simulink model "distance_tracking"  (R2018b)
settings: Solver=ode8  StartTime=0.0  StopTime=20  FixedStep=0.02  RelTol=1e-3
settings Model: Creator=suvo.ganguli  LastModifiedBy=suvo.ganguli

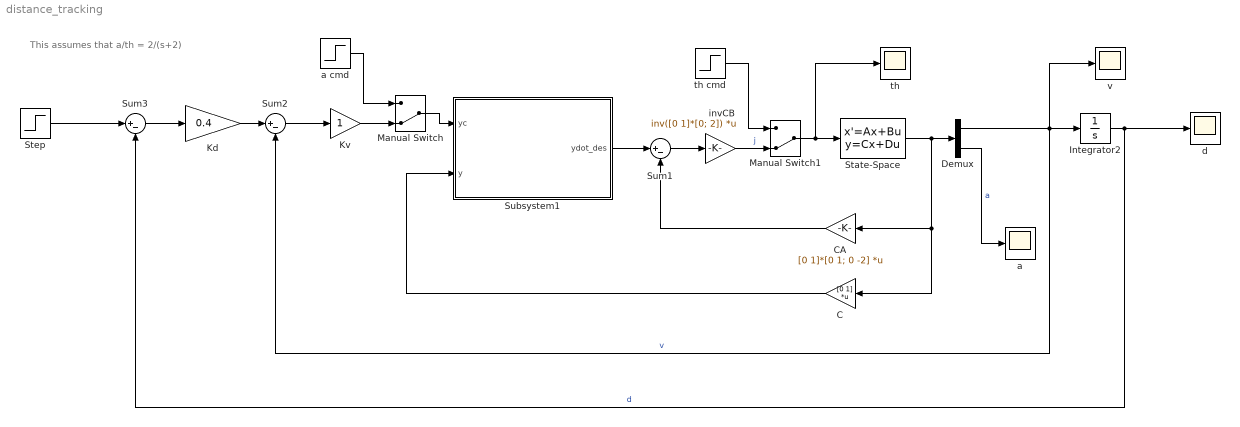
== system distance_tracking ==
  note: This assumes that a/th = 2/(s+2)
  C : Gain  Gain=[0 1]  Multiplication=Matrix(K*u)
  CA : Gain  Gain=[0 1]*[0 1; 0 -2]  Multiplication=Matrix(K*u)
  Demux : Demux  Outputs=2
  Integrator2 : Integrator
  Kd : Gain  Gain=0.4
  Kv : Gain
  Manual Switch : ManualSwitch  CurrentSetting=0
  Manual Switch1 : ManualSwitch  CurrentSetting=0
  State-Space : StateSpace  A=[0 1;0 -2]  B=[0; 2]  C=[1 0;0 1]  D=[0; 0]  InitialCondition=0
  Step : Step  SampleTime=0
  Subsystem1 : Subsystem
  Sum1 : Sum  Inputs=|+-
  Sum2 : Sum  Inputs=|+-
  Sum3 : Sum  Inputs=|+-
  a : Scope
  a cmd : Step  SampleTime=0
  d : Scope
  invCB : Gain  Gain=inv([0 1]*[0; 2])  Multiplication=Matrix(K*u)
  th : Scope
  th cmd : Step  SampleTime=0
  v : Scope
  wires:
  Demux/1 -> v/1, Sum2/2, Integrator2/1  "v"
  Integrator2/1 -> d/1, Sum3/2  "d"
  Sum1/1 -> invCB/1
  CA/1 -> Sum1/2
  State-Space/1 -> CA/1, C/1, Demux/1
  Demux/2 -> a/1  "a"
  C/1 -> Subsystem1/2(y)
  Subsystem1/1(ydot_des) -> Sum1/1
  Sum2/1 -> Kv/1
  Step/1 -> Sum3/1
  Kd/1 -> Sum2/1
  Sum3/1 -> Kd/1
  Kv/1 -> Manual Switch/2
  Manual Switch/1 -> Subsystem1/1(yc)
  a cmd/1 -> Manual Switch/1
  invCB/1 -> Manual Switch1/2  "j"
  Manual Switch1/1 -> th/1, State-Space/1
  th cmd/1 -> Manual Switch1/1

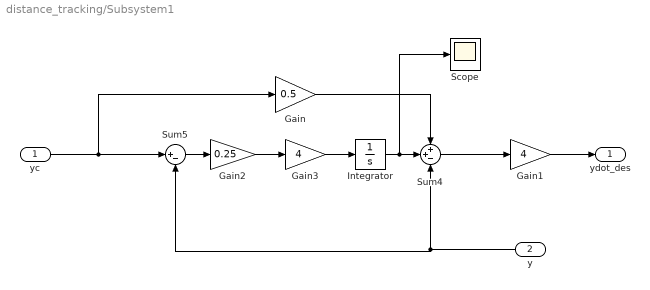
== system distance_tracking/Subsystem1 ==
  yc : Inport
  y : Inport  Port=2
  Gain : Gain  Gain=0.5
  Gain1 : Gain  Gain=4
  Gain2 : Gain  Gain=0.25
  Gain3 : Gain  Gain=4
  Integrator : Integrator
  Scope : Scope
  Sum4 : Sum  Inputs=++-
  Sum5 : Sum  Inputs=|+-
  ydot_des : Outport
  wires:
  Gain3/1 -> Integrator/1
  Sum4/1 -> Gain1/1
  Gain2/1 -> Gain3/1
  Sum5/1 -> Gain2/1
  yc/1 -> Gain/1, Sum5/1
  Integrator/1 -> Scope/1, Sum4/2
  Gain/1 -> Sum4/1
  y/1 -> Sum5/2, Sum4/3
  Gain1/1 -> ydot_des/1
